simulink model "MotionController"  (R2025b)
settings: Solver=FixedStepDiscrete  StartTime=0.0  StopTime=10.0  RelTol=1e-3
settings Model: DataDictionary=embeddedBoard_common.sldd  Creator=rpumpo  LastModifiedBy=rpumpo
settings OptimizationCC: DefaultParameterBehavior=Inlined  UseFloatMulNetSlope=on  EnhancedBackFolding=on  PassReuseOutputArgsAs=Individual arguments  ZeroExternalMemoryAtStartup=off  ZeroInternalMemoryAtStartup=off  OptimizeBlockOrder=speed  DifferentSizesBufferReuse=on  OptimizationCustomize=off  EfficientTunableParamExpr=on
settings DebuggingCC: MultiTaskRateTransMsg=warning  ParameterTunabilityLossMsg=error
settings HardwareCC: ProdBitPerPointer=32.0  ProdBitPerSizeT=32.0  ProdBitPerPtrDiffT=32.0  ProdLargestAtomicInteger=Long  ProdLargestAtomicFloat=Double  ProdWordSize=32.0  ProdHWDeviceType=ARM Compatible->ARM Cortex-M
settings SFSimCC: MATLABDynamicMemAlloc=off
settings RTWCC: SystemTargetFile=ert.tlc  TemplateMakefile=ert_default_tmf  TargetLang=C++  Description=Embedded Coder
settings CodeAppCC: ForceParamTrailComments=on  IgnoreCustomStorageClasses=off  MaxIdLength=60.0  OperatorAnnotations=on  SimulinkDataObjDesc=on  SFDataObjDesc=on  InsertBlockDesc=on
settings ERTTargetCC: RootIOFormat=Structure reference  ERTCustomFileTemplate=example_file_process.tlc  DynamicArrayContainerType=coder::array  TargetLangStandard=C++20 (ISO)  CodeReplacementLibrary=iCubTech  GenerateSampleERTMain=on  CodeInterfacePackaging=C++ class  SubcomponentCodeInterfacePackaging=C++ class

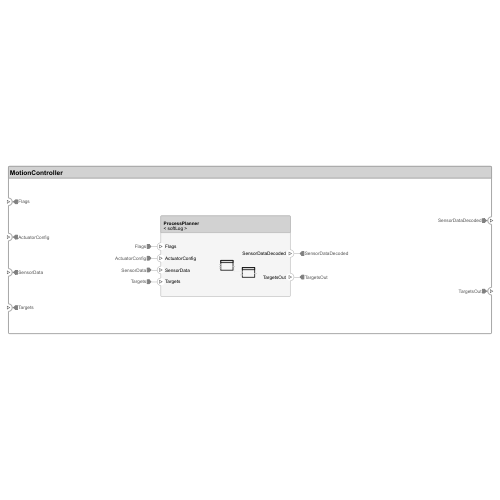
[thumbnail: Simulink's stored preview of the top-level diagram]
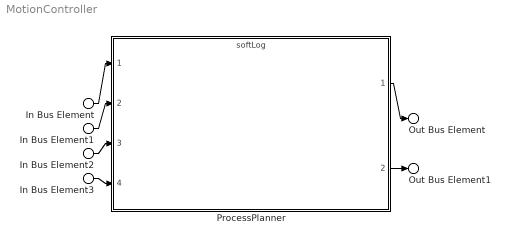
== system MotionController ==
  In Bus Element : Inport  PortName=Flags
  In Bus Element1 : Inport  Port=2  PortName=ActuatorConfig
  In Bus Element2 : Inport  Port=3  PortName=SensorData
  In Bus Element3 : Inport  Port=4  PortName=Targets
  ProcessPlanner : ModelReference  ModelNameDialog=softLog.slx  SimulationMode=Normal  ScheduleRates=on  ModelReferenceVersion=1.74
      settings: PortSchema="{\"entries\":[{\"content\":{\"headerSize\":38,\"margin\":15,\"minimumSpacing\":25,\"sides\":[{\"content\":{\"connectorIds\":[\"In1\",\"In2\",\"In3\",\"In4\"]},\"type\":\"ConnectorPlacement.EquallySpacedRectSide\",\"uuid\":\"5bc97249-f5b2-494b-970a-de3b3bfd1883\"},{\"content\":{\"connectorIds\":[\"Out1\",\"Out2\"],\"side\":\"RIGHT\"},\"type\":\"ConnectorPlacement.EquallySpacedRectSide\",\"uuid\":\"c27ffe8a-4f1e-4977-8b42-d9f4b26c99eb\"},{\"content\":{\"side\":\"TOP\"},\"type\":\"ConnectorPlacement.EquallySpacedRectSide\",\"uuid\":\"ea9c3efe-70a2-4d08-a1da-b2e728a33970\"}]},\"type\":\"ConnectorPlacement.EquallySpacedConnector\",\"uuid\":\"8d7bebf6-8f7c-4b76-a6d3-5057827f12fc\"}],\"packageUris\":[\"http://schema.mathworks.com/mf0/Connector/R2020b\"],\"version\":\"1.0\"}"
  Out Bus Element : Outport  PortName=SensorDataDecoded
  Out Bus Element1 : Outport  Port=2  PortName=TargetsOut
  wires:
  In Bus Element/1 -> ProcessPlanner/1
  In Bus Element1/1 -> ProcessPlanner/2
  In Bus Element2/1 -> ProcessPlanner/3
  In Bus Element3/1 -> ProcessPlanner/4
  ProcessPlanner/1 -> Out Bus Element/1
  ProcessPlanner/2 -> Out Bus Element1/1
